simulink model "problem5"  (R2020a)
settings: Solver=VariableStepAuto  StartTime=0.0  StopTime=10.0  RelTol=1e-3
model workspace (MAT data in the model file):
  R = 10
  c = 1e-05
values from neighbouring files (symbols this model uses):
  q = i*2*10^-3    [intialcondition.m]
settings Model: Creator=Jake  LastModifiedBy=Jake

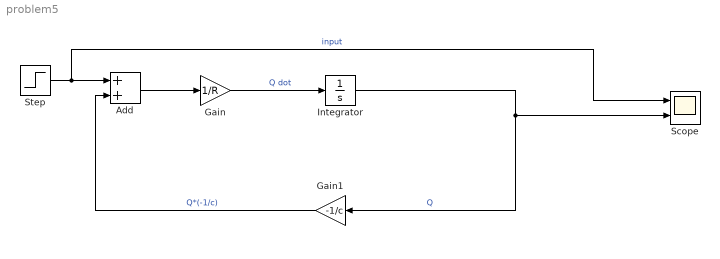
== system problem5 ==
  Add : Sum
  Gain : Gain  Gain=1/R
  Gain1 : Gain  Gain=-1/c
  Integrator : Integrator  InitialCondition=q
  Scope : Scope  NumInputPorts=2
  Step : Step  SampleTime=0
  wires:
  Gain/1 -> Integrator/1  "Q dot"
  Gain1/1 -> Add/2  "Q*(-1/c)"
  Add/1 -> Gain/1
  Step/1 -> Scope/1, Add/1  "input"
  Integrator/1 -> Scope/2, Gain1/1  "Q"
